simulink model "task_2_scheme"  (R2024a)
settings: Solver=VariableStepAuto  StartTime=0.0  StopTime=10.0  RelTol=1e-3
settings Model: Creator=alexe  LastModifiedBy=alexe

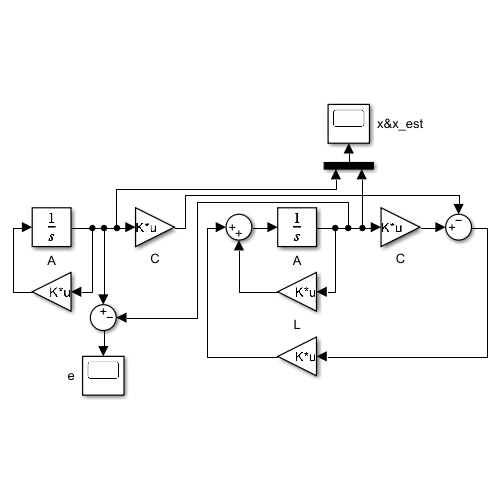
[thumbnail: Simulink's stored preview of the top-level diagram]
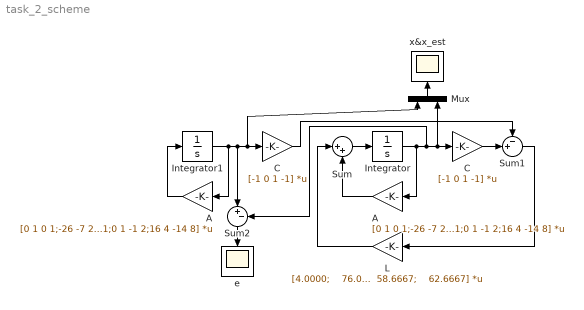
== system task_2_scheme ==
  A : Gain  Gain=[0 1 0 1;-26 -7 20 -11;0 1 -1 2;16 4 -14 8]  Multiplication=Matrix(K*u)
  C : Gain  Gain=[-1 0 1 -1]  Multiplication=Matrix(K*u)
  Integrator : Integrator  InitialCondition=[2;0;0;-1]
  Integrator1 : Integrator  InitialCondition=[1;1;1;1]
  L : Gain  Gain=|  Multiplication=Matrix(K*u)
      | [4.0000;
      |    76.0000;
      |    58.6667;
      |    62.6667]
  Mux : Mux  Inputs=2
  Sum : Sum  Inputs=|++
  Sum1 : Sum  Inputs=-+|
  Sum2 : Sum  Inputs=|+-
  e : Scope
  x&x_est : Scope
  А : Gain  Gain=[0 1 0 1;-26 -7 20 -11;0 1 -1 2;16 4 -14 8]  Multiplication=Matrix(K*u)
  С : Gain  Gain=[-1 0 1 -1]  Multiplication=Matrix(K*u)
  wires:
  Integrator/1 -> C/1, Mux/2, Sum2/2, A/1
  A/1 -> Sum/2
  C/1 -> Sum1/2
  С/1 -> Sum1/1
  Sum1/1 -> L/1
  Integrator1/1 -> С/1, Mux/1, Sum2/1, А/1
  А/1 -> Integrator1/1
  L/1 -> Sum/1
  Sum/1 -> Integrator/1
  Sum2/1 -> e/1
  Mux/1 -> x&x_est/1
